simulink library "Actuators_Block"  (Simulink 8.8)
settings: Solver=VariableStepAuto  StartTime=0.0  StopTime=10.0  RelTol=1e-3
undefined symbols (not defined in the file): CRM
libraries: lib_Sim_CRM x10
settings Model: Creator=cava_da  LastModifiedBy=cava_da

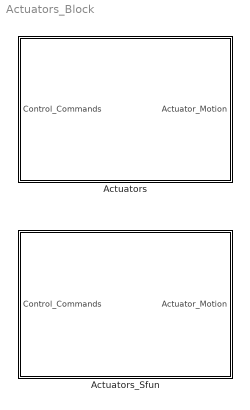
== system Actuators_Block ==
  Actuators : Subsystem
  Actuators_Sfun : Subsystem

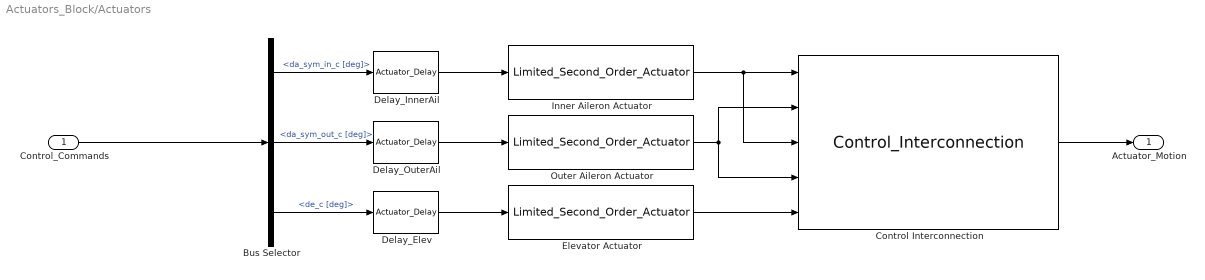
== system Actuators_Block/Actuators ==
  Control_Commands : Inport
  Bus Selector : BusSelector  OutputSignals=da_sym_in_c [deg],da_sym_out_c [deg],de_c [deg]
  Control Interconnection : lib_Sim_CRM/Control_Interconnection
  Delay_Elev : lib_Sim_CRM/Actuator_Delay  Act_Delay=CRM.Actuators.Global_Delay
  Delay_InnerAil : lib_Sim_CRM/Actuator_Delay  Act_Delay=CRM.Actuators.Global_Delay
  Delay_OuterAil : lib_Sim_CRM/Actuator_Delay  Act_Delay=CRM.Actuators.Global_Delay
  Elevator Actuator : lib_Sim_CRM/Limited_Second_Order_Actuator  actuatorName=CRM.Actuators.Elevator
  Inner Aileron Actuator : lib_Sim_CRM/Limited_Second_Order_Actuator  actuatorName=CRM.Actuators.InnerAileron
  Outer Aileron Actuator : lib_Sim_CRM/Limited_Second_Order_Actuator  actuatorName=CRM.Actuators.OuterAileron
  Actuator_Motion : Outport
  wires:
  Inner Aileron Actuator/1 -> Control Interconnection/1, Control Interconnection/3
  Outer Aileron Actuator/1 -> Control Interconnection/4, Control Interconnection/2
  Elevator Actuator/1 -> Control Interconnection/5
  Bus Selector/1 -> Delay_InnerAil/1  "<da_sym_in_c [deg]>"
  Control Interconnection/1 -> Actuator_Motion/1
  Bus Selector/3 -> Delay_Elev/1  "<de_c [deg]>"
  Bus Selector/2 -> Delay_OuterAil/1  "<da_sym_out_c [deg]>"
  Control_Commands/1 -> Bus Selector/1
  Delay_Elev/1 -> Elevator Actuator/1
  Delay_InnerAil/1 -> Inner Aileron Actuator/1
  Delay_OuterAil/1 -> Outer Aileron Actuator/1

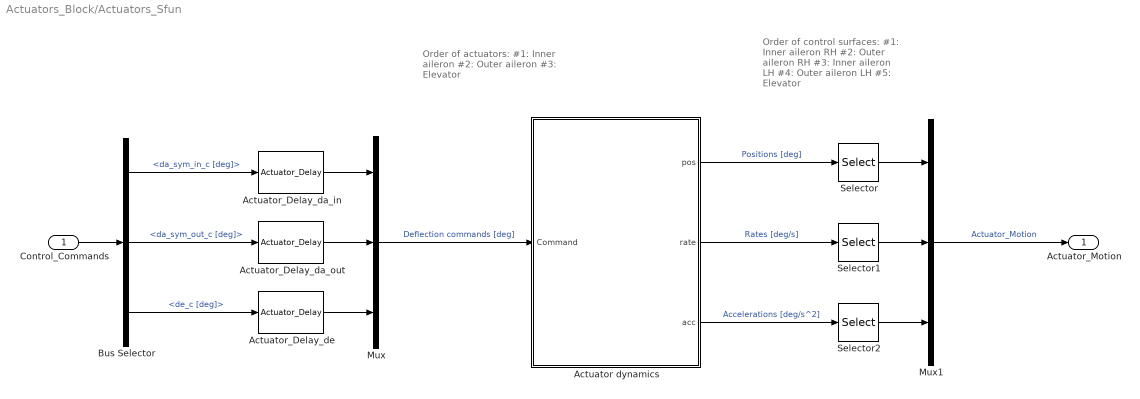
== system Actuators_Block/Actuators_Sfun ==
  note: Order of control surfaces:
      | #1: Inner aileron RH
      | #2: Outer aileron RH
      | #3: Inner aileron LH
      | #4: Outer aileron LH
      | #5: Elevator
  note: Order of actuators:
      | #1: Inner aileron
      | #2: Outer aileron
      | #3: Elevator
  Control_Commands : Inport
  Actuator dynamics : Subsystem
  Actuator_Delay_da_in : lib_Sim_CRM/Actuator_Delay  Act_Delay=CRM.Actuators.Global_Delay
  Actuator_Delay_da_out : lib_Sim_CRM/Actuator_Delay  Act_Delay=CRM.Actuators.Global_Delay
  Actuator_Delay_de : lib_Sim_CRM/Actuator_Delay  Act_Delay=CRM.Actuators.Global_Delay
  Bus Selector : BusSelector  OutputSignals=da_sym_in_c [deg],da_sym_out_c [deg],de_c [deg]
  Mux : Mux  Inputs=3
  Mux1 : Mux  Inputs=3
  Selector : Selector  InputPortWidth=3  IndexOptions=Index vector (dialog)  Indices=[1 2 1 2 3]  OutputSizes=1
  Selector1 : Selector  InputPortWidth=3  IndexOptions=Index vector (dialog)  Indices=[1 2 1 2 3]  OutputSizes=1
  Selector2 : Selector  InputPortWidth=3  IndexOptions=Index vector (dialog)  Indices=[1 2 1 2 3]  OutputSizes=1
  Actuator_Motion : Outport
  wires:
  Control_Commands/1 -> Bus Selector/1
  Actuator dynamics/3(acc) -> Selector2/1  "Accelerations [deg/s^2]"
  Selector/1 -> Mux1/1
  Mux/1 -> Actuator dynamics/1(Command)  "Deflection commands [deg]"
  Selector1/1 -> Mux1/2
  Selector2/1 -> Mux1/3
  Mux1/1 -> Actuator_Motion/1  "Actuator_Motion"
  Bus Selector/2 -> Actuator_Delay_da_out/1  "<da_sym_out_c [deg]>"
  Bus Selector/1 -> Actuator_Delay_da_in/1  "<da_sym_in_c [deg]>"
  Bus Selector/3 -> Actuator_Delay_de/1  "<de_c [deg]>"
  Actuator dynamics/1(pos) -> Selector/1  "Positions [deg]"
  Actuator dynamics/2(rate) -> Selector1/1  "Rates [deg/s]"
  Actuator_Delay_da_in/1 -> Mux/1
  Actuator_Delay_da_out/1 -> Mux/2
  Actuator_Delay_de/1 -> Mux/3

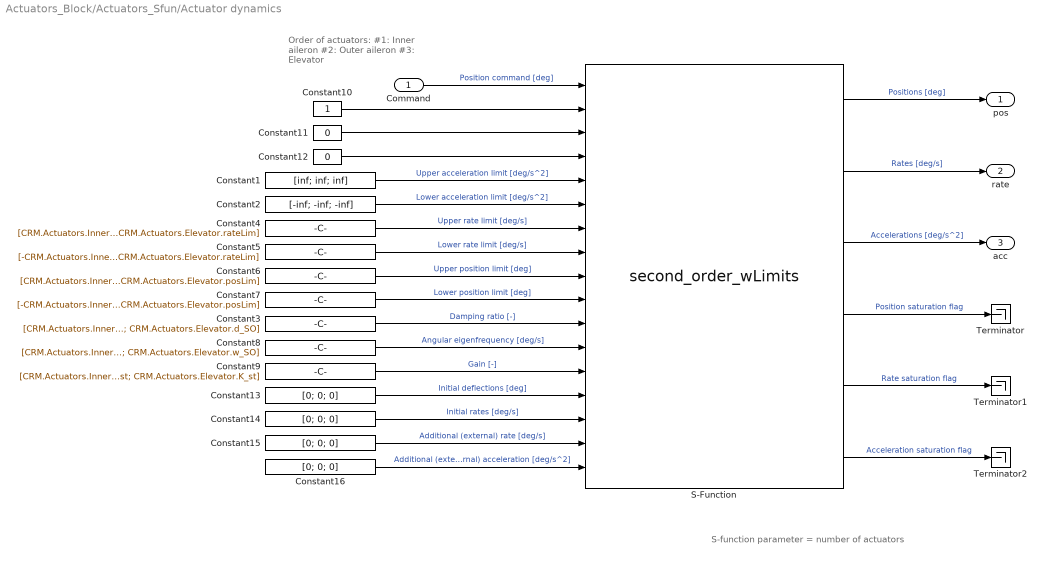
== system Actuators_Block/Actuators_Sfun/Actuator dynamics ==
  note: S-function parameter = number of actuators
  note: Order of actuators:
      | #1: Inner aileron
      | #2: Outer aileron
      | #3: Elevator
  Command : Inport
  Constant1 : Constant  Value=[inf; inf; inf]
  Constant10 : Constant  OutDataTypeStr=boolean
  Constant11 : Constant  Value=0  OutDataTypeStr=boolean
  Constant12 : Constant  Value=0  OutDataTypeStr=boolean
  Constant{13..16} (4 alike) : Constant  Value=[0; 0; 0]
  Constant2 : Constant  Value=[-inf; -inf; -inf]
  Constant3 : Constant  Value=[CRM.Actuators.InnerAileron.d_SO; CRM.Actuators.OuterAileron.d_SO; CRM.Actuators.Elevator.d_SO]
  Constant4 : Constant  Value=[CRM.Actuators.InnerAileron.rateLim; CRM.Actuators.OuterAileron.rateLim; CRM.Actuators.Elevator.rateLim]
  Constant5 : Constant  Value=[-CRM.Actuators.InnerAileron.rateLim; -CRM.Actuators.OuterAileron.rateLim; -CRM.Actuators.Elevator.rateLim]
  Constant6 : Constant  Value=[CRM.Actuators.InnerAileron.posLim; CRM.Actuators.OuterAileron.posLim; CRM.Actuators.Elevator.posLim]
  Constant7 : Constant  Value=[-CRM.Actuators.InnerAileron.posLim; -CRM.Actuators.OuterAileron.posLim; -CRM.Actuators.Elevator.posLim]
  Constant8 : Constant  Value=[CRM.Actuators.InnerAileron.w_SO; CRM.Actuators.OuterAileron.w_SO; CRM.Actuators.Elevator.w_SO]
  Constant9 : Constant  Value=[CRM.Actuators.InnerAileron.K_st; CRM.Actuators.OuterAileron.K_st; CRM.Actuators.Elevator.K_st]
  S-Function : S-Function  FunctionName=second_order_wLimits  Parameters=3  SFunctionDeploymentMode=off  EnableBusSupport=off
      mask Display:
      | port_label('input',1,'command');
      | port_label('input',2,'run');
      | port_label('input',3,'reset');
      | port_label('input',4,'Trim_Lin');
      | port_label('input',5,'acc_lim_up');
      | port_label('input',6,'acc_lim_low');
      | port_label('input',7,'rate_lim_up');
      | port_label('input',8,'rate_lim_low');
      | port_label('input',9,'pos_lim_up');
      | port_label('input',10,'pos_lim_low');
      | port_label('input',11,'xi');
      | port_label('input',12,'omega');
      | port_label('input',13,'K');
      | port_label('input',14,'x0');
      | port_label('input',15,'xdot0');
      | port_label('input',16,'delta_x_dot');
      | port_label('input',17,'delta_x_dotdot');
      | 
      | port_label('output',1,'x');
      | port_label('output',2,'xdot');
      | port_label('output',3,'xdotdot');
      | port_label('output',4,'sat_pos');
      | port_label('output',5,'sat_rate');
      | port_label('output',6,'sat_acc');
  Terminator : Terminator
  Terminator1 : Terminator
  Terminator2 : Terminator
  pos : Outport
  rate : Outport  Port=2
  acc : Outport  Port=3
  wires:
  Command/1 -> S-Function/1  "Position command [deg]"
  Constant12/1 -> S-Function/4
  Constant11/1 -> S-Function/3
  Constant1/1 -> S-Function/5  "Upper acceleration limit [deg/s^2]"
  Constant2/1 -> S-Function/6  "Lower acceleration limit [deg/s^2]"
  Constant4/1 -> S-Function/7  "Upper rate limit [deg/s]"
  Constant5/1 -> S-Function/8  "Lower rate limit [deg/s]"
  Constant3/1 -> S-Function/11  "Damping ratio [-]"
  Constant9/1 -> S-Function/13  "Gain [-]"
  Constant13/1 -> S-Function/14  "Initial deflections [deg]"
  Constant8/1 -> S-Function/12  "Angular eigenfrequency [deg/s]"
  Constant14/1 -> S-Function/15  "Initial rates [deg/s]"
  S-Function/1 -> pos/1  "Positions [deg]"
  S-Function/2 -> rate/1  "Rates [deg/s]"
  S-Function/3 -> acc/1  "Accelerations [deg/s^2]"
  S-Function/4 -> Terminator/1  "Position saturation flag"
  S-Function/5 -> Terminator1/1  "Rate saturation flag"
  S-Function/6 -> Terminator2/1  "Acceleration saturation flag"
  Constant15/1 -> S-Function/16  "Additional (external) rate [deg/s]"
  Constant16/1 -> S-Function/17  "Additional (external) acceleration [deg/s^2]"
  Constant6/1 -> S-Function/9  "Upper position limit [deg]"
  Constant7/1 -> S-Function/10  "Lower position limit [deg]"
  Constant10/1 -> S-Function/2
